simulink model "bh_SIM_7dof_car_active_suspension"  (R2022b)
settings: Solver=ode23t  StartTime=0.0  StopTime=10  FixedStep=0.0005  MaxStep=0.001  RelTol=1e-5
undefined symbols (not defined in the file): Continuous, K, OBJ_car_params, Time, X, Y, Z
libraries: sm_lib x23, nesl_utility x4, ctrlSharedLib x1
settings Model: Creator=bhorton  LastModifiedBy=bhorton
settings SolverCC: ZeroCrossAlgorithm=Adaptive
settings DebuggingCC: UnconnectedInputMsg=warning  UnconnectedOutputMsg=warning  UnconnectedLineMsg=warning
settings ModelReferenceCC: EnableRefExpFcnMdlSchedulingChecks=on
settings RTWCC: DLArmComputeVersion=19.05
settings ExplorerConfigSet: InternalSimMechanicsExplorerSettings="<ExplorerConfiguration><canonicalview>default</canonicalview><AnimationSetting><BasePlaybackSpeed>1.0</BasePlaybackSpeed><PlaybackSpeedFactor>1.0</PlaybackSpeedFactor></AnimationSetting><TilePanel><TileInfo><Tiles Columns=\"2\" Count=\"3\" Rows=\"2\"><Column Weight=\"0.4994\"/><Column Weight=\"0.5006\"/><Row Weight=\"0.4993\"/><Row Weight=\"0.5007\"/><Tile Height=\"1\" Width=\"2\" X=\"0\" Y=\"0\"/><Tile Height=\"1\" Width=\"1\" X=\"0\" Y=\"1\"/><Tile Height=\"1\" Width=\"1\" X=\"1\" Y=\"1\"/></Tiles></TileInfo><SceneInfo><SceneViewer><BGColor><R>0.60000002384185791</R><G>0.60000002384185791</G><B>0.60000002384185791</B></BGColor><Camera><DoPerspective>off</DoPerspective><Position><X>28.1684565527861146</X><Y>9.37690846949945644</Y><Z>23.0019248509705427</Z></Position><Center><X>8.88421556953053937</X><Y>0.438838580194179317</Y><Z>-4.64373243439162042</Z></Center><Up><X>-0.185673330126828295</X><Y>0.96548958646651295</Y><Z>-0.182634259941381938</Z></Up><ViewLimDist>1</ViewLimDist><YLim>3.64885946251190196</YLim><XLim>10.9300677112347469</XLim></Camera></SceneViewer><SceneViewer><BGColor><R>0.60000002384185791</R><G>0.60000002384185791</G><B>0.60000002384185791</B></BGColor><Camera><DoPerspective>off</DoPerspective><Position><X>5.74701636142130656</X><Y>11.5370316322497803</Y><Z>70.170564057313058</Z></Position><Center><X>1.87189459127800673</X><Y>1.93296934541278587</Y><Z>-0.938513511499806441</Z></Center><Up><X>-0.0228131350943184333</X><Y>0.990908416802929626</Y><Z>-0.132589857742894418</Z></Up><ViewLimDist>1</ViewLimDist><YLim>3.40641172776440104</YLim><XLim>5.04056870527299949</XLim></Camera></SceneViewer><SceneViewer><BGColor><R>0.60000002384185791</R><G>0.60000002384185791</G><B>0.60000002384185791</B></BGColor><Camera><DoPerspective>off</DoPerspective><Position><X>16.559571799394174</X><Y>1.27394383122949439</Y><Z>-2.29291646985018405</Z></Position><Center><X>1.86700752803715142</X><Y>-0.342587176142176597</Y><Z>-3.18464415250598165</Z></Center><Up><X>-0.109797444713875203</X><Y>0.993927323497863835</Y><Z>0.0072798858972461869</Z></Up><ViewLimDist>1</ViewLimDist><YLim>2.89568809729259158</YLim><XLim>4.29135758562730896</XLim></Camera></SceneViewer></SceneInfo></TilePanel><MechEditorPanel><Cameras/><GfxPanelCameraMap/><VideoCreator><PlaybackSpeedRatio>1.0</PlaybackSpeedRatio><FrameRate>30</FrameRate><VideoFormat>MPEG-4</VideoFormat><FrameSize>[400 400]</FrameSize></VideoCreator></MechEditorPanel></ExplorerConfiguration>"

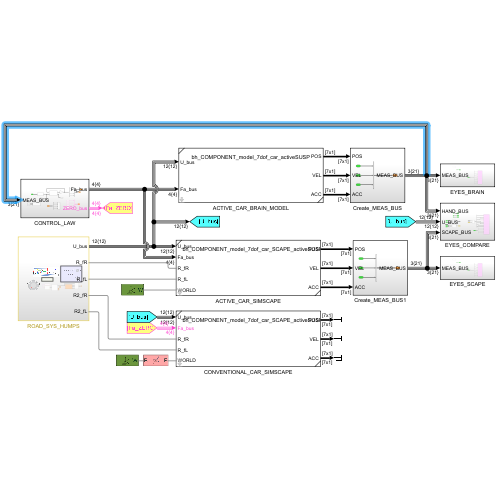
[thumbnail: Simulink's stored preview of the top-level diagram]
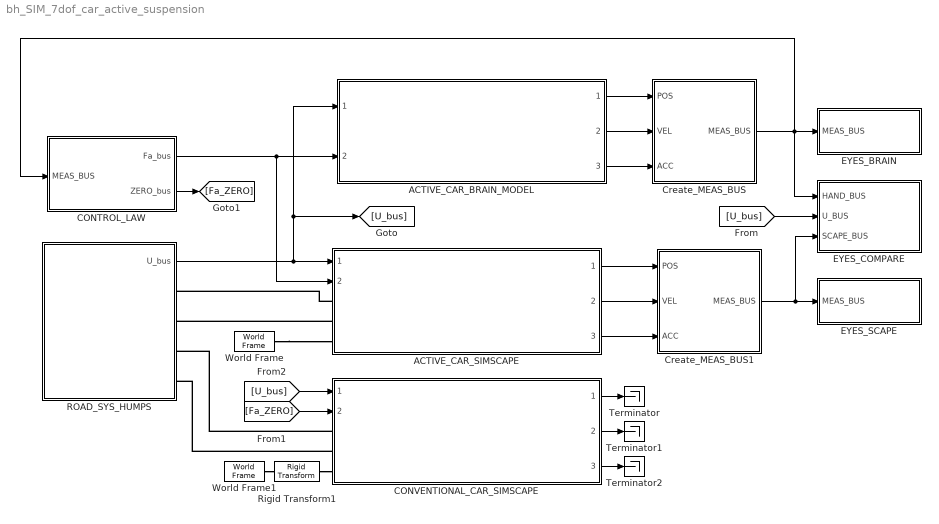
== system bh_SIM_7dof_car_active_suspension ==
  ACTIVE_CAR_BRAIN_MODEL : Subsystem  ReferencedSubsystem=bh_COMPONENT_model_7dof_car_activeSUSP  L_b=OBJ_car_params.L_b  L_f=OBJ_car_params.L_f  L_R=OBJ_car_params.L_R  L_L=OBJ_car_params.L_L  m_c=OBJ_car_params.m_c  I_cZ=OBJ_car_params.I_cZ  I_cX=OBJ_car_params.I_cX  m_bR=OBJ_car_params.m_bR  m_fR=OBJ_car_params.m_fR  m_bL=OBJ_car_params.m_bL  m_fL=OBJ_car_params.m_fL  k_bR=OBJ_car_params.k_bR  k_fR=OBJ_car_params.k_fR  k_bL=OBJ_car_params.k_bL  k_fL=OBJ_car_params.k_fL  k_bRG=OBJ_car_params.k_bRG  k_fRG=OBJ_car_params.k_fRG  k_bLG=OBJ_car_params.k_bLG  k_fLG=OBJ_car_params.k_fLG  c_bR=OBJ_car_params.c_bR  c_fR=OBJ_car_params.c_fR  c_bL=OBJ_car_params.c_bL  c_fL=OBJ_car_params.c_fL  c_bRG=OBJ_car_params.c_bRG  c_fRG=OBJ_car_params.c_fRG  c_bLG=OBJ_car_params.c_bLG  c_fLG=OBJ_car_params.c_fLG  IC_pos=OBJ_car_params.IC_pos  IC_vel=OBJ_car_params.IC_vel
  ACTIVE_CAR_SIMSCAPE : Subsystem  ReferencedSubsystem=bh_COMPONENT_model_7dof_car_SCAPE_activeSUSP  L_b=OBJ_car_params.L_b  L_f=OBJ_car_params.L_f  L_R=OBJ_car_params.L_R  L_L=OBJ_car_params.L_L  m_c=OBJ_car_params.m_c  I_cZ=OBJ_car_params.I_cZ  I_cX=OBJ_car_params.I_cX  m_bR=OBJ_car_params.m_bR  m_fR=OBJ_car_params.m_fR  m_bL=OBJ_car_params.m_bL  m_fL=OBJ_car_params.m_fL  k_bR=OBJ_car_params.k_bR  k_fR=OBJ_car_params.k_fR  k_bL=OBJ_car_params.k_bL  k_fL=OBJ_car_params.k_fL  k_bRG=OBJ_car_params.k_bRG  k_fRG=OBJ_car_params.k_fRG  k_bLG=OBJ_car_params.k_bLG  k_fLG=OBJ_car_params.k_fLG  c_bR=OBJ_car_params.c_bR  c_fR=OBJ_car_params.c_fR  c_bL=OBJ_car_params.c_bL  c_fL=OBJ_car_params.c_fL  c_bRG=OBJ_car_params.c_bRG  c_fRG=OBJ_car_params.c_fRG  c_bLG=OBJ_car_params.c_bLG  c_fLG=OBJ_car_params.c_fLG  IC_pos=OBJ_car_params.IC_pos  IC_vel=OBJ_car_params.IC_vel
  CONTROL_LAW : Subsystem
  CONVENTIONAL_CAR_SIMSCAPE : Subsystem  ReferencedSubsystem=bh_COMPONENT_model_7dof_car_SCAPE_activeSUSP  L_b=OBJ_car_params.L_b  L_f=OBJ_car_params.L_f  L_R=OBJ_car_params.L_R  L_L=OBJ_car_params.L_L  m_c=OBJ_car_params.m_c  I_cZ=OBJ_car_params.I_cZ  I_cX=OBJ_car_params.I_cX  m_bR=OBJ_car_params.m_bR  m_fR=OBJ_car_params.m_fR  m_bL=OBJ_car_params.m_bL  m_fL=OBJ_car_params.m_fL  k_bR=OBJ_car_params.k_bR  k_fR=OBJ_car_params.k_fR  k_bL=OBJ_car_params.k_bL  k_fL=OBJ_car_params.k_fL  k_bRG=OBJ_car_params.k_bRG  k_fRG=OBJ_car_params.k_fRG  k_bLG=OBJ_car_params.k_bLG  k_fLG=OBJ_car_params.k_fLG  c_bR=OBJ_car_params.c_bR  c_fR=OBJ_car_params.c_fR  c_bL=OBJ_car_params.c_bL  c_fL=OBJ_car_params.c_fL  c_bRG=OBJ_car_params.c_bRG  c_fRG=OBJ_car_params.c_fRG  c_bLG=OBJ_car_params.c_bLG  c_fLG=OBJ_car_params.c_fLG  IC_pos=OBJ_car_params.IC_pos  IC_vel=OBJ_car_params.IC_vel
  Create_MEAS_BUS : Subsystem
  Create_MEAS_BUS1 : Subsystem
  EYES_BRAIN : Subsystem
  EYES_COMPARE : Subsystem
  EYES_SCAPE : Subsystem
  ROAD_SYS_HUMPS : Subsystem
  Rigid Transform1 : sm_lib/Frames and Transforms/Rigid Transform  TranslationMethod=StandardAxis  TranslationStandardOffset=2*(OBJ_car_params.L_R + OBJ_car_params.L_L)  TranslationLengthUnit=m  TranslationStandardAxis=-Z  TranslationCartesianOffset=[0 0 0]  TranslationROffset=0  TranslationROffsetUnits=m  TranslationZOffset=0  TranslationZOffsetUnits=m  TranslationThetaOffset=0  TranslationThetaOffsetUnits=deg  RotationMethod=None  RotationAngleUnits=deg  RotationStandardAxis=+Z  RotationAngle=0.0  RotationArbitraryAxis=[0 0 1]  FollAlignAxisA=+X  BaseAlignAxisA=+Y  FollAlignAxisB=+Y  BaseAlignAxisB=+Z  RotationSequenceAxes=FollowerAxes  RotationSequence=XYX  RotationSequenceAngles=[0 0 0]  RotationSequenceAnglesUnits=deg  RotationMatrix=[1 0 0; 0 1 0; 0 0 1]  Quaternion=[1 0 0 0]
  Terminator : Terminator
  Terminator1 : Terminator
  Terminator2 : Terminator
  World Frame : sm_lib/Frames and Transforms/World Frame
  World Frame1 : sm_lib/Frames and Transforms/World Frame
  wires:
  ACTIVE_CAR_BRAIN_MODEL/1 -> Create_MEAS_BUS/1(POS)
  ACTIVE_CAR_BRAIN_MODEL/2 -> Create_MEAS_BUS/2(VEL)
  ACTIVE_CAR_BRAIN_MODEL/3 -> Create_MEAS_BUS/3(ACC)
  Create_MEAS_BUS/1(MEAS_BUS) -> EYES_COMPARE/1(HAND_BUS), CONTROL_LAW/1(MEAS_BUS), EYES_BRAIN/1(MEAS_BUS)
  ACTIVE_CAR_SIMSCAPE/1 -> Create_MEAS_BUS1/1(POS)
  ACTIVE_CAR_SIMSCAPE/2 -> Create_MEAS_BUS1/2(VEL)
  ACTIVE_CAR_SIMSCAPE/3 -> Create_MEAS_BUS1/3(ACC)
  Create_MEAS_BUS1/1(MEAS_BUS) -> EYES_COMPARE/3(SCAPE_BUS), EYES_SCAPE/1(MEAS_BUS)
  ROAD_SYS_HUMPS/1(U_bus) -> ACTIVE_CAR_BRAIN_MODEL/1, [U_bus], ACTIVE_CAR_SIMSCAPE/1
  [U_bus] -> EYES_COMPARE/2(U_BUS)
  CONTROL_LAW/2(ZERO_bus) -> [Fa_ZERO]
  CONTROL_LAW/1(Fa_bus) -> ACTIVE_CAR_SIMSCAPE/2, ACTIVE_CAR_BRAIN_MODEL/2
  [Fa_ZERO] -> CONVENTIONAL_CAR_SIMSCAPE/2
  [U_bus] -> CONVENTIONAL_CAR_SIMSCAPE/1
  CONVENTIONAL_CAR_SIMSCAPE/1 -> Terminator/1
  CONVENTIONAL_CAR_SIMSCAPE/2 -> Terminator1/1
  CONVENTIONAL_CAR_SIMSCAPE/3 -> Terminator2/1
  connections:
  ACTIVE_CAR_SIMSCAPE/LConn1 -- ROAD_SYS_HUMPS/RConn1
  ACTIVE_CAR_SIMSCAPE/LConn2 -- ROAD_SYS_HUMPS/RConn2
  World Frame1/RConn1 -- Rigid Transform1/LConn1
  Rigid Transform1/RConn1 -- CONVENTIONAL_CAR_SIMSCAPE/LConn3
  World Frame/RConn1 -- ACTIVE_CAR_SIMSCAPE/LConn3
  CONVENTIONAL_CAR_SIMSCAPE/LConn1 -- ROAD_SYS_HUMPS/RConn3
  CONVENTIONAL_CAR_SIMSCAPE/LConn2 -- ROAD_SYS_HUMPS/RConn4

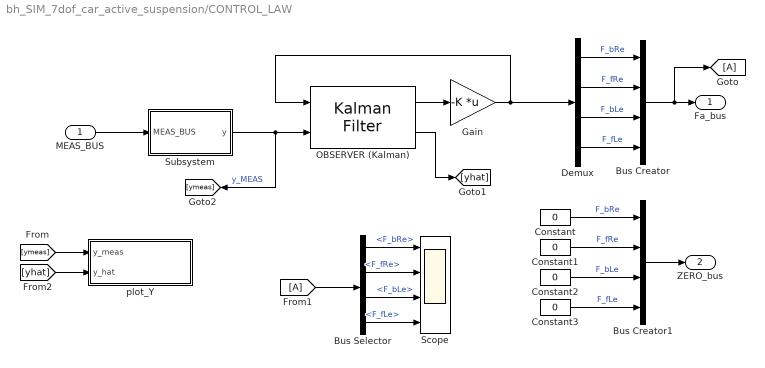
== system bh_SIM_7dof_car_active_suspension/CONTROL_LAW ==
  MEAS_BUS : Inport
  Bus Creator : BusCreator  Inputs=4
  Bus Creator1 : BusCreator  Inputs=4
  Bus Selector : BusSelector  OutputSignals=F_bRe,F_fRe,F_bLe,F_fLe
  Constant{,1..3} (4 alike) : Constant  Value=0
  Demux : Demux
  From1 : From
  Gain : Gain  Gain=-K  Multiplication=Matrix(K*u)
  Goto : Goto
  OBSERVER (Kalman) : ctrlSharedLib/Kalman Filter  TimeDomain=Continuous-Time  UseCurrentEstimator=on  ModelSource=LTI State-Space Variable  ModelSourceVariable=my_sys  A=0.95  B=1  C=1  D=0  NumberOfStates=1  NumberOfInputs=1  NumberOfOutputs=1  InitialEstimateSource=Dialog  X0=0  P0=10  UseK=off  UseGH=off  NumberOfProcessNoiseInputs=1  G=1  TimeInvariantG=on  H=0  TimeInvariantH=on  Q=1e8  TimeInvariantQ=on  R=1  TimeInvariantR=on  N=0  TimeInvariantN=on  AddInputPort=on  AddEnablePort=off  OutputEstimatedY=on  OutputP=off  Ts=-1
  Scope : Scope  NumInputPorts=4
  Subsystem : Subsystem
  plot_Y : Subsystem
  Fa_bus : Outport
  ZERO_bus : Outport  Port=2
  wires:
  MEAS_BUS/1 -> Subsystem/1(MEAS_BUS)
  Gain/1 -> OBSERVER (Kalman)/1, Demux/1
  Subsystem/1(y) -> [ymeas], OBSERVER (Kalman)/2  "y_MEAS"
  OBSERVER (Kalman)/1 -> Gain/1
  Demux/4 -> Bus Creator/4  "F_fLe"
  Demux/3 -> Bus Creator/3  "F_bLe"
  Demux/2 -> Bus Creator/2  "F_fRe"
  Demux/1 -> Bus Creator/1  "F_bRe"
  Bus Creator/1 -> Fa_bus/1, Goto/1
  From1/1 -> Bus Selector/1
  Bus Selector/1 -> Scope/1  "<F_bRe>"
  Bus Selector/2 -> Scope/2  "<F_fRe>"
  Bus Selector/3 -> Scope/3  "<F_bLe>"
  Bus Selector/4 -> Scope/4  "<F_fLe>"
  Bus Creator1/1 -> ZERO_bus/1
  Constant/1 -> Bus Creator1/1  "F_bRe"
  Constant3/1 -> Bus Creator1/4  "F_fLe"
  Constant2/1 -> Bus Creator1/3  "F_bLe"
  Constant1/1 -> Bus Creator1/2  "F_fRe"
  OBSERVER (Kalman)/2 -> [yhat]
  [ymeas] -> plot_Y/1(y_meas)
  [yhat] -> plot_Y/2(y_hat)

== system bh_SIM_7dof_car_active_suspension/Create_MEAS_BUS ==
  POS : Inport
  VEL : Inport  Port=2
  ACC : Inport  Port=3
  Bus Creator : BusCreator  Inputs=3
  MEAS_BUS : Outport
  wires:
  POS/1 -> Bus Creator/1  "POS"
  VEL/1 -> Bus Creator/2  "VEL"
  ACC/1 -> Bus Creator/3  "ACC"
  Bus Creator/1 -> MEAS_BUS/1

== system bh_SIM_7dof_car_active_suspension/Create_MEAS_BUS1 ==
  POS : Inport
  VEL : Inport  Port=2
  ACC : Inport  Port=3
  Bus Creator : BusCreator  Inputs=3
  MEAS_BUS : Outport
  wires:
  POS/1 -> Bus Creator/1  "POS"
  VEL/1 -> Bus Creator/2  "VEL"
  ACC/1 -> Bus Creator/3  "ACC"
  Bus Creator/1 -> MEAS_BUS/1

== system bh_SIM_7dof_car_active_suspension/EYES_BRAIN ==
  note: % NOTE:  the order of the DOF vector is:
      | %          1      2    3     4     5     6     7
      | %      [ y_c, theta, psi, y_bR, y_fR, y_bL, y_fL ]
  MEAS_BUS : Inport
  Bus Selector : BusSelector  OutputSignals=POS
  Demux : Demux  Outputs=7
  Ground : Ground
  HAND_POS : Scope  NumInputPorts=8
  Subsystem : Subsystem  Commented=on
  wires:
  MEAS_BUS/1 -> [MEAS]
  Demux/1 -> HAND_POS/1  "y_c"
  Demux/2 -> HAND_POS/2  "theta"
  Demux/3 -> HAND_POS/3  "psi"
  Ground/1 -> HAND_POS/4
  Demux/4 -> HAND_POS/5  "y_bR"
  Demux/5 -> HAND_POS/6  "y_fR"
  Demux/6 -> HAND_POS/7  "y_bL"
  Demux/7 -> HAND_POS/8  "y_fL"
  [MEAS] -> Bus Selector/1
  Bus Selector/1 -> Demux/1  "<POS>"

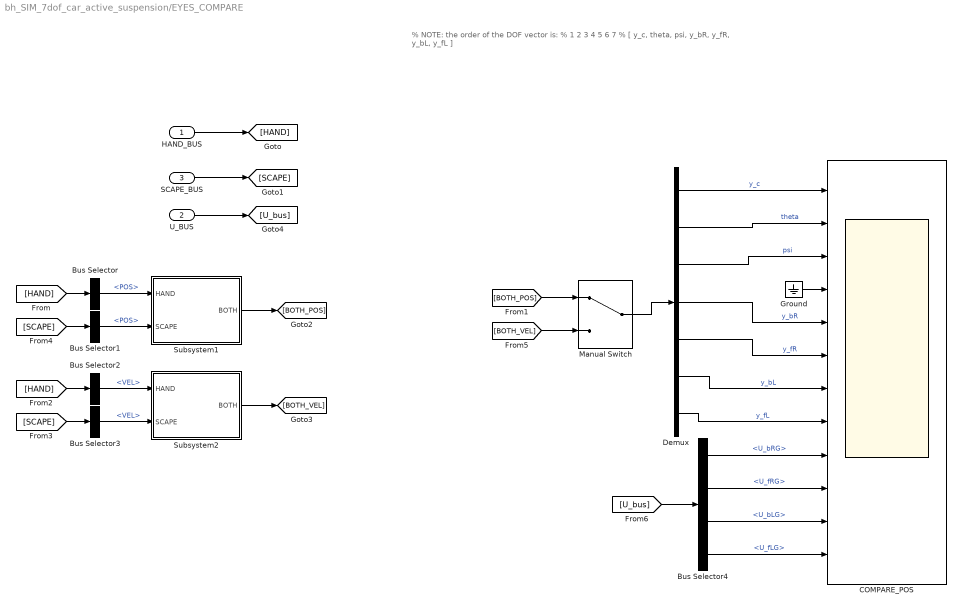
== system bh_SIM_7dof_car_active_suspension/EYES_COMPARE ==
  note: % NOTE:  the order of the DOF vector is:
      | %          1      2    3     4     5     6     7
      | %      [ y_c, theta, psi, y_bR, y_fR, y_bL, y_fL ]
  HAND_BUS : Inport
  U_BUS : Inport  Port=2
  SCAPE_BUS : Inport  Port=3
  Bus Selector : BusSelector  OutputSignals=POS
  Bus Selector1 : BusSelector  OutputSignals=POS
  Bus Selector2 : BusSelector  OutputSignals=VEL
  Bus Selector3 : BusSelector  OutputSignals=VEL
  Bus Selector4 : BusSelector  OutputSignals=U_bRG,U_fRG,U_bLG,U_fLG
  COMPARE_POS : Scope  NumInputPorts=12
  Demux : Demux  Outputs=7
  Ground : Ground
  Manual Switch : ManualSwitch
  Subsystem1 : Subsystem
  Subsystem2 : Subsystem
  wires:
  HAND_BUS/1 -> [HAND]
  Demux/1 -> COMPARE_POS/1  "y_c"
  Demux/2 -> COMPARE_POS/2  "theta"
  Demux/3 -> COMPARE_POS/3  "psi"
  Ground/1 -> COMPARE_POS/4
  Demux/5 -> COMPARE_POS/6  "y_fR"
  Demux/6 -> COMPARE_POS/7  "y_bL"
  Demux/7 -> COMPARE_POS/8  "y_fL"
  SCAPE_BUS/1 -> [SCAPE]
  [HAND] -> Bus Selector/1
  [SCAPE] -> Bus Selector1/1
  Bus Selector/1 -> Subsystem1/1(HAND)  "<POS>"
  Bus Selector1/1 -> Subsystem1/2(SCAPE)  "<POS>"
  Subsystem1/1(BOTH) -> [BOTH_POS]
  [HAND] -> Bus Selector2/1
  Subsystem2/1(BOTH) -> [BOTH_VEL]
  Bus Selector2/1 -> Subsystem2/1(HAND)  "<VEL>"
  Bus Selector3/1 -> Subsystem2/2(SCAPE)  "<VEL>"
  [SCAPE] -> Bus Selector3/1
  Manual Switch/1 -> Demux/1
  [BOTH_VEL] -> Manual Switch/2
  [BOTH_POS] -> Manual Switch/1
  U_BUS/1 -> [U_bus]
  [U_bus] -> Bus Selector4/1
  Bus Selector4/4 -> COMPARE_POS/12  "<U_fLG>"
  Bus Selector4/3 -> COMPARE_POS/11  "<U_bLG>"
  Bus Selector4/2 -> COMPARE_POS/10  "<U_fRG>"
  Bus Selector4/1 -> COMPARE_POS/9  "<U_bRG>"
  Demux/4 -> COMPARE_POS/5  "y_bR"

== system bh_SIM_7dof_car_active_suspension/EYES_SCAPE ==
  note: % NOTE:  the order of the DOF vector is:
      | %          1      2    3     4     5     6     7
      | %      [ y_c, theta, psi, y_bR, y_fR, y_bL, y_fL ]
  MEAS_BUS : Inport
  Bus Selector : BusSelector  OutputSignals=POS
  Demux : Demux  Outputs=7
  Ground : Ground
  SCAPE_POS : Scope  NumInputPorts=8
  Subsystem : Subsystem  Commented=on
  wires:
  MEAS_BUS/1 -> [MEAS]
  Demux/1 -> SCAPE_POS/1  "y_c"
  Demux/2 -> SCAPE_POS/2  "theta"
  Demux/3 -> SCAPE_POS/3  "psi"
  Ground/1 -> SCAPE_POS/4
  Demux/4 -> SCAPE_POS/5  "y_bR"
  Demux/5 -> SCAPE_POS/6  "y_fR"
  Demux/6 -> SCAPE_POS/7  "y_bL"
  Demux/7 -> SCAPE_POS/8  "y_fL"
  [MEAS] -> Bus Selector/1
  Bus Selector/1 -> Demux/1  "<POS>"

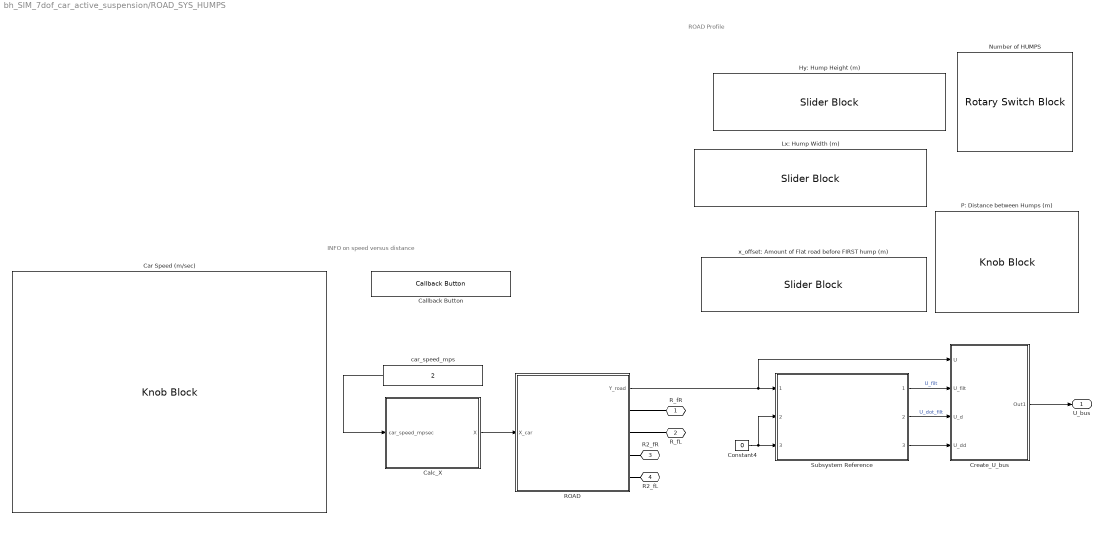
== system bh_SIM_7dof_car_active_suspension/ROAD_SYS_HUMPS ==
  note: INFO on speed versus distance
  note: ROAD Profile
  Calc_X : Subsystem
  Callback Button : CallbackButton  ButtonText=Open XLS file to view
      settings: ClickFcn=winopen bh_speed_vs_distance_explore.xlsx
  Car Speed (m/sec) : KnobBlock  LabelPosition=Hide  ScaleMax=30  TickInterval=1
  Constant4 : Constant  Value=0
  Create_U_bus : Subsystem
  Hy: Hump Height (m) : SliderBlock  LabelPosition=Hide  ScaleMax=0.16
  Lx: Hump Width (m) : SliderBlock  LabelPosition=Hide  ScaleMax=1
  Number of HUMPS : RotarySwitchBlock  LabelPosition=Hide
      settings: Values={{'1', '3', '5', '10', '20', '50', '100'}, [1 3 5 10 20 50 100]}
  P: Distance between Humps (m) : KnobBlock  LabelPosition=Hide
  ROAD : Subsystem  mask{m_Hy=0.16, m_Lx=1, m_P=2, m_x_offset=2, m_Np=5}
      mask prompts: m_Hy "Height of hump (m)"; m_Lx "Length of hump (m)"; m_P "Period of window (m)"; m_x_offset "X direction offset"; m_Np "Number of periods"
      mask init:
      | % create SYS object
      | OBJ = bh_road_hump_A_SYSO("Hy",m_Hy, "Lx",m_Lx, "P",m_P, ...
      |                           "x_offset",m_x_offset, "NUM_PERIODS",m_Np);
      |                       
      | tmp_x = linspace(0,(m_Np*m_P  +  m_x_offset), 1e4);
      | tmp_y = OBJ.get_y(tmp_x);
      | %tmp_z = -2 * ones(size(tmp_x));
      | tmp_z = zeros(size(tmp_x));
      | the_road_XYZ = [ tmp_x(:), tmp_y(:), tmp_z(:) ];
      mask DialogControl Control2 Prompt: Road Profile Parameters
      mask DialogControl Container6 Prompt: Road Profile Parameters
  Subsystem Reference : Subsystem  ReferencedSubsystem=bh_COMPONENT_deriv_est  wn=2*pi*5000  p=1
  car_speed_mps : Constant  Value=2
  x_offset: Amount of Flat road before FIRST hump (m) : SliderBlock  LabelPosition=Hide  ScaleMax=10
  R_fR : PMIOPort  Side=Right
  R_fL : PMIOPort  Port=2  Side=Right
  R2_fR : PMIOPort  Port=3  Side=Right
  R2_fL : PMIOPort  Port=4  Side=Right
  U_bus : Outport
  wires:
  Create_U_bus/1(Out1) -> U_bus/1
  ROAD/1(Y_road) -> Create_U_bus/1(U), Subsystem Reference/1
  Constant4/1 -> Subsystem Reference/2, Subsystem Reference/3
  Subsystem Reference/3 -> Create_U_bus/4(U_dd)
  Subsystem Reference/2 -> Create_U_bus/3(U_d)  "U_dot_filt"
  Subsystem Reference/1 -> Create_U_bus/2(U_filt)  "U_filt"
  Calc_X/1(X) -> ROAD/1(X_car)
  car_speed_mps/1 -> Calc_X/1(car_speed_mpsec)
  connections:
  R_fL/RConn1 -- ROAD/RConn2
  ROAD/RConn1 -- R_fR/RConn1
  ROAD/RConn3 -- R2_fR/RConn1
  ROAD/RConn4 -- R2_fL/RConn1

== system bh_SIM_7dof_car_active_suspension/CONTROL_LAW/Subsystem ==
  note: $X^T =\left\lbrack \begin{array}{ccccccc} y_c & \theta & \psi & y_{\mathrm{bR}} & y_{\mathrm{fR}} & y_{\mathrm{bL}} & y_{\mathrm{fL}} \end{array}\right\rbrack \\ Z=\left\lbrack \begin{array}{c} \dot{X} \\ X \end{array}\right\rbrack \\ y={\left\lbrack \begin{array}{cccccc} y_c & \theta & \psi & \dot{y_c } & \dot{\theta} & \dot{\psi} \end{array}\right\rbrack }^T$
  MEAS_BUS : Inport
  Bus Selector : BusSelector  OutputSignals=VEL,POS
  Constant4 : Constant  Value="[8,9,10,  1,2,3]"
  Selector : Selector  InputPortWidth=14  IndexOptions=Index vector (port)  Indices=[1 3]  OutputSizes=1
  Vector Concatenate : Concatenate
  y : Outport
  wires:
  Bus Selector/1 -> Vector Concatenate/1  "<VEL>"
  MEAS_BUS/1 -> Bus Selector/1
  Bus Selector/2 -> Vector Concatenate/2  "<POS>"
  Constant4/1 -> Selector/2  "F_fLe"
  Vector Concatenate/1 -> Selector/1  "Z"
  Selector/1 -> y/1

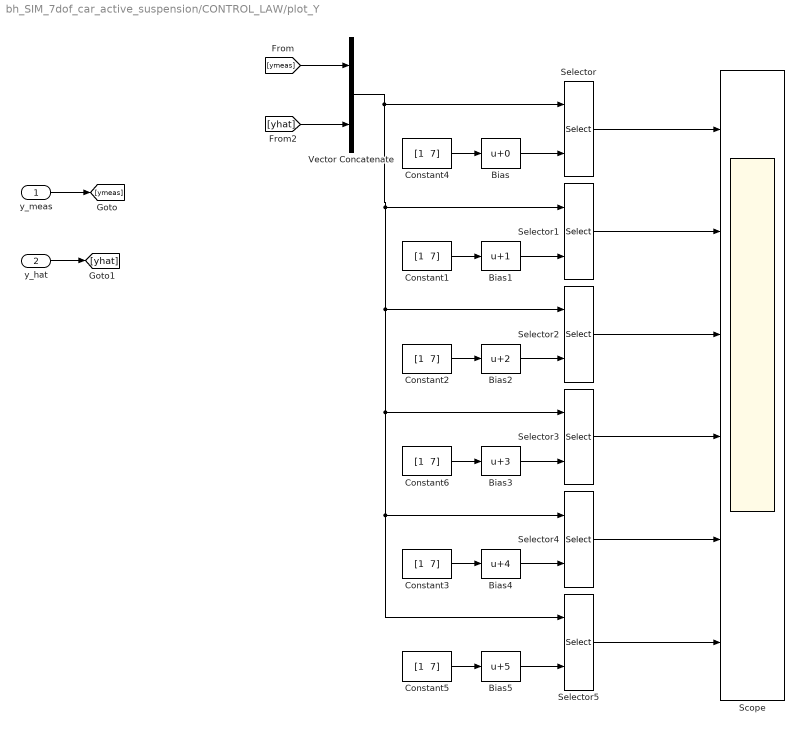
== system bh_SIM_7dof_car_active_suspension/CONTROL_LAW/plot_Y ==
  y_meas : Inport
  y_hat : Inport  Port=2
  Bias : Bias  SaturateOnIntegerOverflow=off
  Bias1 : Bias  Bias=1  SaturateOnIntegerOverflow=off
  Bias2 : Bias  Bias=2  SaturateOnIntegerOverflow=off
  Bias3 : Bias  Bias=3  SaturateOnIntegerOverflow=off
  Bias4 : Bias  Bias=4  SaturateOnIntegerOverflow=off
  Bias5 : Bias  Bias=5  SaturateOnIntegerOverflow=off
  Constant{1..6} (6 alike) : Constant  Value="[1  7]"
  Scope : Scope  NumInputPorts=6
  Selector{,1..5} (6 alike) : Selector  InputPortWidth=12  IndexOptions=Index vector (port)  Indices=[1 3]  OutputSizes=1
  Vector Concatenate : Concatenate
  wires:
  y_meas/1 -> [ymeas]
  y_hat/1 -> [yhat]
  [ymeas] -> Vector Concatenate/1
  [yhat] -> Vector Concatenate/2
  Constant4/1 -> Bias/1
  Bias/1 -> Selector/2
  Selector/1 -> Scope/1
  Bias1/1 -> Selector1/2
  Constant1/1 -> Bias1/1
  Selector1/1 -> Scope/2
  Bias2/1 -> Selector2/2
  Constant2/1 -> Bias2/1
  Selector2/1 -> Scope/3
  Bias3/1 -> Selector3/2
  Constant3/1 -> Bias4/1
  Bias4/1 -> Selector4/2
  Vector Concatenate/1 -> Selector3/1, Selector5/1, Selector4/1, Selector2/1, Selector1/1, Selector/1
  Constant6/1 -> Bias3/1
  Bias5/1 -> Selector5/2
  Constant5/1 -> Bias5/1
  Selector3/1 -> Scope/4
  Selector4/1 -> Scope/5
  Selector5/1 -> Scope/6

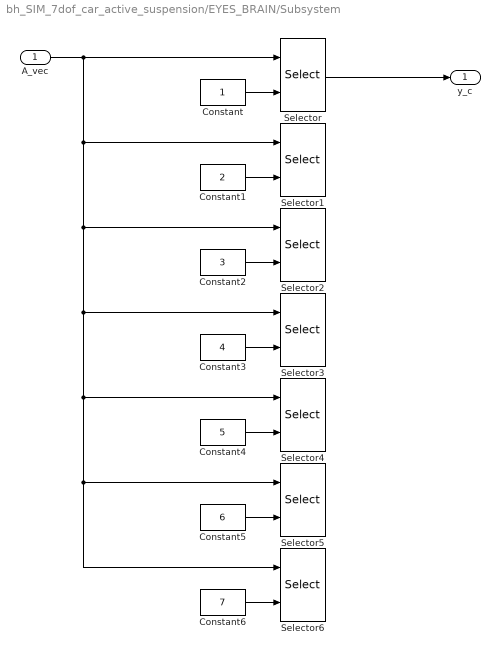
== system bh_SIM_7dof_car_active_suspension/EYES_BRAIN/Subsystem ==
  A_vec : Inport
  Constant : Constant
  Constant1 : Constant  Value=2
  Constant2 : Constant  Value=3
  Constant3 : Constant  Value=4
  Constant4 : Constant  Value=5
  Constant5 : Constant  Value=6
  Constant6 : Constant  Value=7
  Selector{,1..6} (7 alike) : Selector  InputPortWidth=7  IndexOptions=Index vector (port)  Indices=1  OutputSizes=1
  y_c : Outport
  wires:
  Constant/1 -> Selector/2
  Constant1/1 -> Selector1/2
  Constant2/1 -> Selector2/2
  Constant3/1 -> Selector3/2
  Constant4/1 -> Selector4/2
  Constant5/1 -> Selector5/2
  Constant6/1 -> Selector6/2
  A_vec/1 -> Selector1/1, Selector2/1, Selector3/1, Selector4/1, Selector5/1, Selector6/1, Selector/1
  Selector/1 -> y_c/1

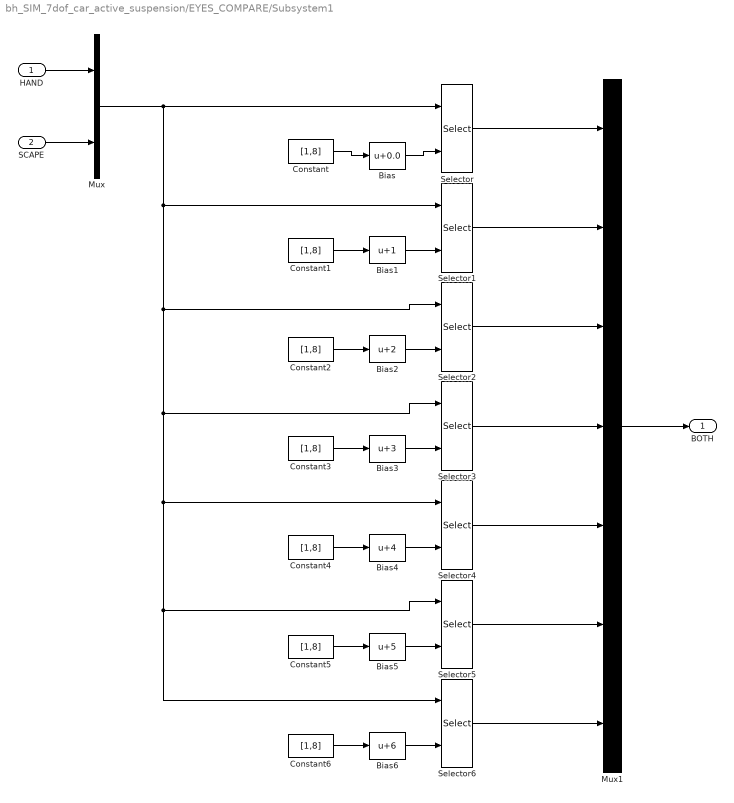
== system bh_SIM_7dof_car_active_suspension/EYES_COMPARE/Subsystem1 ==
  HAND : Inport
  SCAPE : Inport  Port=2
  Bias : Bias  Bias=0.0  SaturateOnIntegerOverflow=off
  Bias1 : Bias  Bias=1  SaturateOnIntegerOverflow=off
  Bias2 : Bias  Bias=2  SaturateOnIntegerOverflow=off
  Bias3 : Bias  Bias=3  SaturateOnIntegerOverflow=off
  Bias4 : Bias  Bias=4  SaturateOnIntegerOverflow=off
  Bias5 : Bias  Bias=5  SaturateOnIntegerOverflow=off
  Bias6 : Bias  Bias=6  SaturateOnIntegerOverflow=off
  Constant{,1..6} (7 alike) : Constant  Value=[1,8]
  Mux : Mux  Inputs=2
  Mux1 : Mux  Inputs=7
  Selector{,1..6} (7 alike) : Selector  InputPortWidth=14  IndexOptions=Index vector (port)  Indices=[1 3]  OutputSizes=1
  BOTH : Outport
  wires:
  SCAPE/1 -> Mux/2
  HAND/1 -> Mux/1
  Constant/1 -> Bias/1
  Bias/1 -> Selector/2
  Selector/1 -> Mux1/1
  Selector1/1 -> Mux1/2
  Bias1/1 -> Selector1/2
  Constant1/1 -> Bias1/1
  Constant2/1 -> Bias2/1
  Bias2/1 -> Selector2/2
  Selector2/1 -> Mux1/3
  Bias3/1 -> Selector3/2
  Constant3/1 -> Bias3/1
  Selector3/1 -> Mux1/4
  Constant4/1 -> Bias4/1
  Bias4/1 -> Selector4/2
  Selector4/1 -> Mux1/5
  Constant5/1 -> Bias5/1
  Bias5/1 -> Selector5/2
  Constant6/1 -> Bias6/1
  Bias6/1 -> Selector6/2
  Mux/1 -> Selector1/1, Selector2/1, Selector3/1, Selector4/1, Selector5/1, Selector6/1, Selector/1
  Selector5/1 -> Mux1/6
  Selector6/1 -> Mux1/7
  Mux1/1 -> BOTH/1

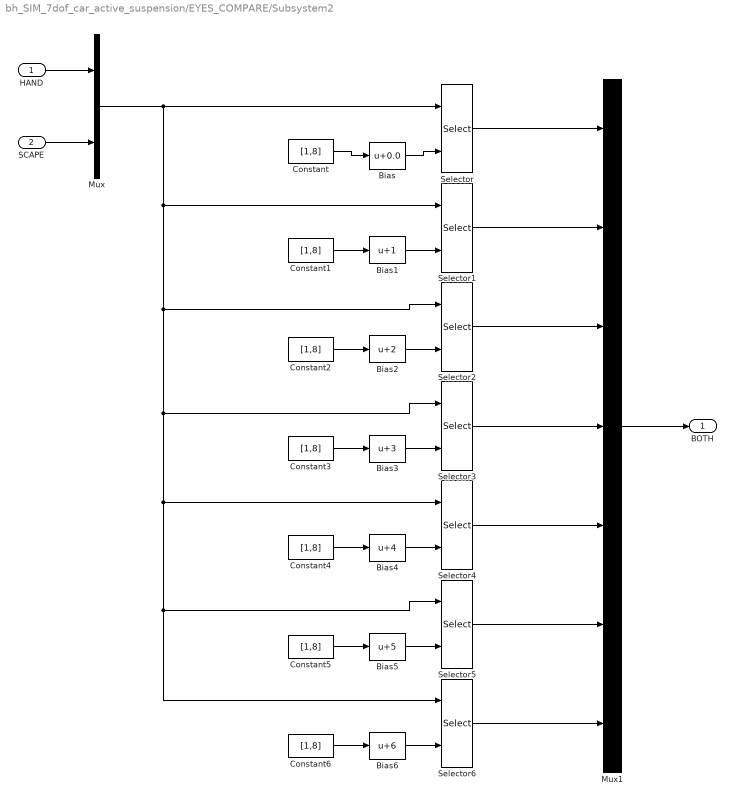
== system bh_SIM_7dof_car_active_suspension/EYES_COMPARE/Subsystem2 ==
  HAND : Inport
  SCAPE : Inport  Port=2
  Bias : Bias  Bias=0.0  SaturateOnIntegerOverflow=off
  Bias1 : Bias  Bias=1  SaturateOnIntegerOverflow=off
  Bias2 : Bias  Bias=2  SaturateOnIntegerOverflow=off
  Bias3 : Bias  Bias=3  SaturateOnIntegerOverflow=off
  Bias4 : Bias  Bias=4  SaturateOnIntegerOverflow=off
  Bias5 : Bias  Bias=5  SaturateOnIntegerOverflow=off
  Bias6 : Bias  Bias=6  SaturateOnIntegerOverflow=off
  Constant{,1..6} (7 alike) : Constant  Value=[1,8]
  Mux : Mux  Inputs=2
  Mux1 : Mux  Inputs=7
  Selector{,1..6} (7 alike) : Selector  InputPortWidth=14  IndexOptions=Index vector (port)  Indices=[1 3]  OutputSizes=1
  BOTH : Outport
  wires:
  SCAPE/1 -> Mux/2
  HAND/1 -> Mux/1
  Constant/1 -> Bias/1
  Bias/1 -> Selector/2
  Selector/1 -> Mux1/1
  Selector1/1 -> Mux1/2
  Bias1/1 -> Selector1/2
  Constant1/1 -> Bias1/1
  Constant2/1 -> Bias2/1
  Bias2/1 -> Selector2/2
  Selector2/1 -> Mux1/3
  Bias3/1 -> Selector3/2
  Constant3/1 -> Bias3/1
  Selector3/1 -> Mux1/4
  Constant4/1 -> Bias4/1
  Bias4/1 -> Selector4/2
  Selector4/1 -> Mux1/5
  Constant5/1 -> Bias5/1
  Bias5/1 -> Selector5/2
  Constant6/1 -> Bias6/1
  Bias6/1 -> Selector6/2
  Mux/1 -> Selector1/1, Selector2/1, Selector3/1, Selector4/1, Selector5/1, Selector6/1, Selector/1
  Selector5/1 -> Mux1/6
  Selector6/1 -> Mux1/7
  Mux1/1 -> BOTH/1

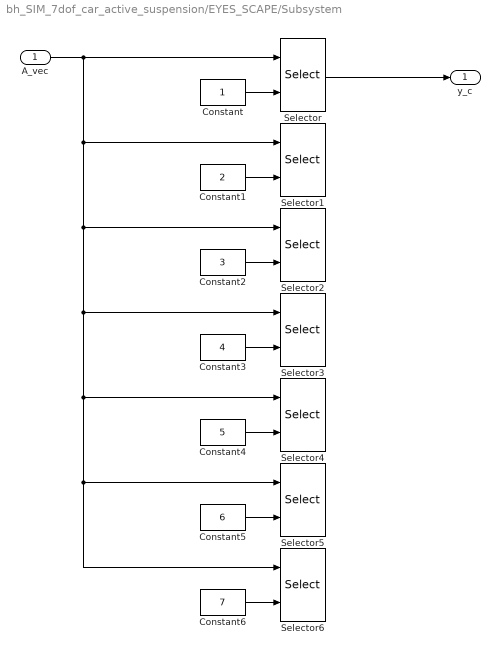
== system bh_SIM_7dof_car_active_suspension/EYES_SCAPE/Subsystem ==
  A_vec : Inport
  Constant : Constant
  Constant1 : Constant  Value=2
  Constant2 : Constant  Value=3
  Constant3 : Constant  Value=4
  Constant4 : Constant  Value=5
  Constant5 : Constant  Value=6
  Constant6 : Constant  Value=7
  Selector{,1..6} (7 alike) : Selector  InputPortWidth=7  IndexOptions=Index vector (port)  Indices=1  OutputSizes=1
  y_c : Outport
  wires:
  Constant/1 -> Selector/2
  Constant1/1 -> Selector1/2
  Constant2/1 -> Selector2/2
  Constant3/1 -> Selector3/2
  Constant4/1 -> Selector4/2
  Constant5/1 -> Selector5/2
  Constant6/1 -> Selector6/2
  A_vec/1 -> Selector1/1, Selector2/1, Selector3/1, Selector4/1, Selector5/1, Selector6/1, Selector/1
  Selector/1 -> y_c/1

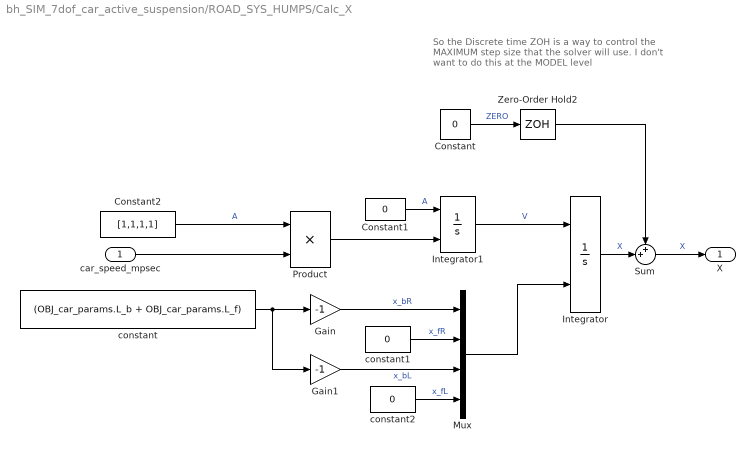
== system bh_SIM_7dof_car_active_suspension/ROAD_SYS_HUMPS/Calc_X ==
  note: So the Discrete time ZOH is a way to control
      | the MAXIMUM step size that the solver will use.
      |
      | I don't want to do this at the MODEL level
  car_speed_mpsec : Inport
  Constant : Constant  Value=0
  Constant1 : Constant  Value=0
  Constant2 : Constant  Value=[1,1,1,1]
  Gain : Gain  Gain=-1
  Gain1 : Gain  Gain=-1
  Integrator : Integrator  InitialConditionSource=external
  Integrator1 : Integrator  InitialConditionSource=external
  Mux : Mux
  Product : Product
  Sum : Sum  Inputs=++|
  Zero-Order Hold2 : ZeroOrderHold  SampleTime=1/1000
      settings: AttributesFormatString=dT =%<SampleTime>
  constant : Constant  Value=(OBJ_car_params.L_b + OBJ_car_params.L_f)
  constant1 : Constant  Value=0
  constant2 : Constant  Value=0
  X : Outport
  wires:
  Integrator1/1 -> Integrator/1  "V"
  Zero-Order Hold2/1 -> Sum/1
  car_speed_mpsec/1 -> Product/2
  Integrator/1 -> Sum/2  "X"
  Constant/1 -> Zero-Order Hold2/1  "ZERO"
  Mux/1 -> Integrator/2
  Constant1/1 -> Integrator1/1  "A"
  constant/1 -> Gain1/1, Gain/1
  constant2/1 -> Mux/4  "x_fL"
  Gain1/1 -> Mux/3  "x_bL"
  constant1/1 -> Mux/2  "x_fR"
  Gain/1 -> Mux/1  "x_bR"
  Sum/1 -> X/1  "X"
  Constant2/1 -> Product/1  "A"
  Product/1 -> Integrator1/2

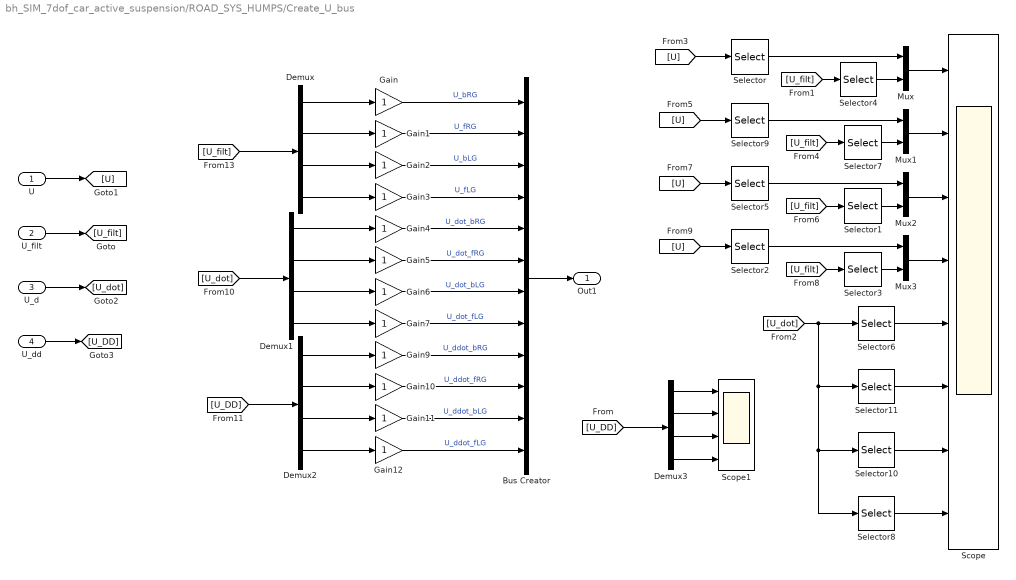
== system bh_SIM_7dof_car_active_suspension/ROAD_SYS_HUMPS/Create_U_bus ==
  U : Inport
  U_filt : Inport  Port=2
  U_d : Inport  Port=3
  U_dd : Inport  Port=4
  Bus Creator : BusCreator  Inputs=12
  Demux{,1..3} (4 alike) : Demux
  Gain{,1..7,9..12} (12 alike) : Gain
  Mux{,1..3} (4 alike) : Mux  Inputs=2
  Scope : Scope  NumInputPorts=8
  Scope1 : Scope  NumInputPorts=4
  Selector : Selector  InputPortWidth=4  IndexOptions=Index vector (dialog)  Indices=1  OutputSizes=1
  Selector1 : Selector  InputPortWidth=4  IndexOptions=Index vector (dialog)  Indices=3  OutputSizes=1
  Selector10 : Selector  InputPortWidth=4  IndexOptions=Index vector (dialog)  Indices=3  OutputSizes=1
  Selector11 : Selector  InputPortWidth=4  IndexOptions=Index vector (dialog)  Indices=2  OutputSizes=1
  Selector2 : Selector  InputPortWidth=4  IndexOptions=Index vector (dialog)  Indices=4  OutputSizes=1
  Selector3 : Selector  InputPortWidth=4  IndexOptions=Index vector (dialog)  Indices=4  OutputSizes=1
  Selector4 : Selector  InputPortWidth=4  IndexOptions=Index vector (dialog)  Indices=1  OutputSizes=1
  Selector5 : Selector  InputPortWidth=4  IndexOptions=Index vector (dialog)  Indices=3  OutputSizes=1
  Selector6 : Selector  InputPortWidth=4  IndexOptions=Index vector (dialog)  Indices=1  OutputSizes=1
  Selector7 : Selector  InputPortWidth=4  IndexOptions=Index vector (dialog)  Indices=2  OutputSizes=1
  Selector8 : Selector  InputPortWidth=4  IndexOptions=Index vector (dialog)  Indices=4  OutputSizes=1
  Selector9 : Selector  InputPortWidth=4  IndexOptions=Index vector (dialog)  Indices=2  OutputSizes=1
  Out1 : Outport
  wires:
  Demux/1 -> Gain/1
  [U_dot] -> Selector11/1, Selector10/1, Selector8/1, Selector6/1
  Gain9/1 -> Bus Creator/9  "U_ddot_bRG"
  Gain10/1 -> Bus Creator/10  "U_ddot_fRG"
  Gain1/1 -> Bus Creator/2  "U_fRG"
  Demux/2 -> Gain1/1
  Mux/1 -> Scope/1
  Demux/3 -> Gain2/1
  Demux2/2 -> Gain10/1
  Demux1/4 -> Gain7/1
  Demux3/3 -> Scope1/3
  Gain4/1 -> Bus Creator/5  "U_dot_bRG"
  Demux1/2 -> Gain5/1
  Demux1/3 -> Gain6/1
  Selector6/1 -> Scope/5
  Gain7/1 -> Bus Creator/8  "U_dot_fLG"
  Demux2/1 -> Gain9/1
  Gain5/1 -> Bus Creator/6  "U_dot_fRG"
  Demux1/1 -> Gain4/1
  [U_filt] -> Selector1/1
  Selector3/1 -> Mux3/2
  Gain2/1 -> Bus Creator/3  "U_bLG"
  Demux/4 -> Gain3/1
  [U] -> Selector2/1
  Gain3/1 -> Bus Creator/4  "U_fLG"
  Selector10/1 -> Scope/7
  Selector7/1 -> Mux1/2
  Selector4/1 -> Mux/2
  Selector11/1 -> Scope/6
  Gain/1 -> Bus Creator/1  "U_bRG"
  Mux2/1 -> Scope/3
  Mux1/1 -> Scope/2
  Mux3/1 -> Scope/4
  Selector5/1 -> Mux2/1
  [U] -> Selector/1
  Selector8/1 -> Scope/8
  Gain6/1 -> Bus Creator/7  "U_dot_bLG"
  Selector2/1 -> Mux3/1
  [U] -> Selector5/1
  Selector1/1 -> Mux2/2
  Selector9/1 -> Mux1/1
  Demux3/2 -> Scope1/2
  [U_filt] -> Selector4/1
  [U_filt] -> Selector7/1
  Selector/1 -> Mux/1
  Demux3/1 -> Scope1/1
  Gain12/1 -> Bus Creator/12  "U_ddot_fLG"
  [U] -> Selector9/1
  Bus Creator/1 -> Out1/1
  Demux3/4 -> Scope1/4
  Demux2/4 -> Gain12/1
  [U_DD] -> Demux3/1
  Gain11/1 -> Bus Creator/11  "U_ddot_bLG"
  [U_filt] -> Selector3/1
  Demux2/3 -> Gain11/1
  U/1 -> [U]
  U_filt/1 -> [U_filt]
  U_d/1 -> [U_dot]
  U_dd/1 -> [U_DD]
  [U_dot] -> Demux1/1
  [U_DD] -> Demux2/1
  [U_filt] -> Demux/1

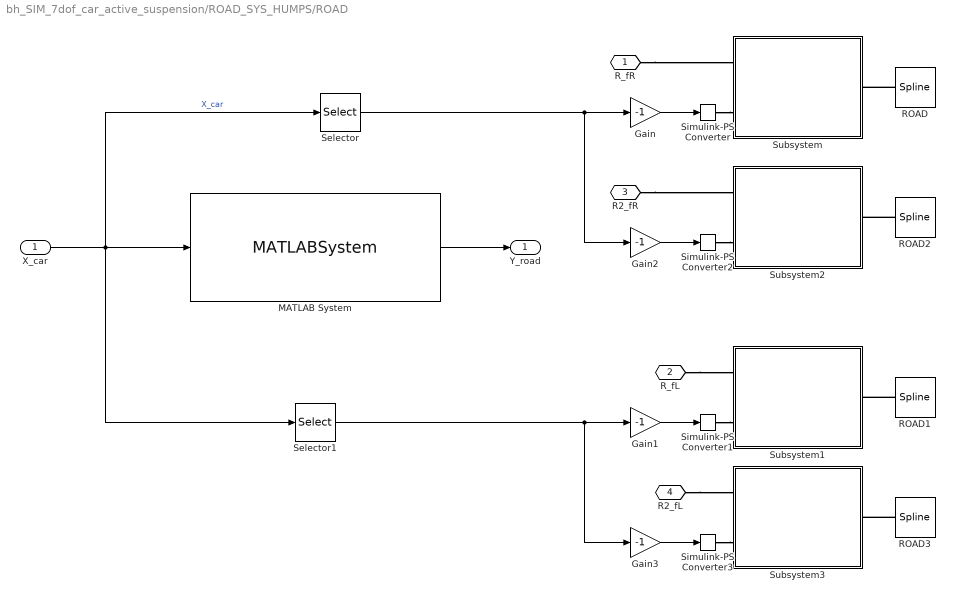
== system bh_SIM_7dof_car_active_suspension/ROAD_SYS_HUMPS/ROAD ==
  X_car : Inport
  Gain{,1..3} (4 alike) : Gain  Gain=-1
  MATLAB System : MATLABSystem  System=bh_road_hump_A_SYSO  Hy=m_Hy  Lx=m_Lx  P=m_P  x_offset=m_x_offset  NUM_PERIODS=m_Np  SimulateUsing=Interpreted execution
      mask Type: bh_road_hump_A_SYSO
      mask Display:
      | disp('bh_road_hump_A_SYSO');
      | port_label('input',1,'X_car');
      | port_label('output',1,'Y_road');
  ROAD : sm_lib/Curves and Surfaces/Spline  GraphicAmbientColor=[0.15 0.15 0.15 1.0]  GraphicDiffuseColor=[0.2 1.0 0.2]  DataPoints=the_road_XYZ  DataPointsUnits=m  GraphicEmissiveColor=[0.0 0.0 0.0 1.0]  EndConditionType=Natural  MarkerShape=Sphere  MarkerSize=10  GraphicType=FromGeometry  GraphicOpacity=1.0  GraphicShininess=75  GraphicSpecularColor=[0.5 0.5 0.5 1.0]  GraphicVisPropType=SimpleVisualProperties
  ROAD1 : sm_lib/Curves and Surfaces/Spline  GraphicAmbientColor=[0.15 0.15 0.15 1.0]  GraphicDiffuseColor=[0.2 1.0 0.2]  DataPoints=the_road_XYZ  DataPointsUnits=m  GraphicEmissiveColor=[0.0 0.0 0.0 1.0]  EndConditionType=Natural  MarkerShape=Sphere  MarkerSize=10  GraphicType=FromGeometry  GraphicOpacity=1.0  GraphicShininess=75  GraphicSpecularColor=[0.5 0.5 0.5 1.0]  GraphicVisPropType=SimpleVisualProperties
  ROAD2 : sm_lib/Curves and Surfaces/Spline  GraphicAmbientColor=[0.15 0.15 0.15 1.0]  GraphicDiffuseColor=[1, 0.6, 0.6]  DataPoints=the_road_XYZ  DataPointsUnits=m  GraphicEmissiveColor=[0.0 0.0 0.0 1.0]  EndConditionType=Natural  MarkerShape=Sphere  MarkerSize=10  GraphicType=FromGeometry  GraphicOpacity=1.0  GraphicShininess=75  GraphicSpecularColor=[0.5 0.5 0.5 1.0]  GraphicVisPropType=SimpleVisualProperties
  ROAD3 : sm_lib/Curves and Surfaces/Spline  GraphicAmbientColor=[0.15 0.15 0.15 1.0]  GraphicDiffuseColor=[1.0 0.6 0.6]  DataPoints=the_road_XYZ  DataPointsUnits=m  GraphicEmissiveColor=[0.0 0.0 0.0 1.0]  EndConditionType=Natural  MarkerShape=Sphere  MarkerSize=10  GraphicType=FromGeometry  GraphicOpacity=1.0  GraphicShininess=75  GraphicSpecularColor=[0.5 0.5 0.5 1.0]  GraphicVisPropType=SimpleVisualProperties
  Selector : Selector  InputPortWidth=4  IndexOptions=Index vector (dialog)  Indices=2  OutputSizes=1
  Selector1 : Selector  InputPortWidth=4  IndexOptions=Index vector (dialog)  Indices=4  OutputSizes=1
  Simulink-PS Converter{,1..3} (4 alike) : nesl_utility/Simulink-PS Converter  PhysicalDomain=network_engine_domain  SubClassName=ps_input  LeftPortType=input  RightPortType=output  PseudoPeriodic=off  Frequencies=[]  NoiseDistribution=none  NoiseParameters=[]  Unit=m  AffineConversion=off  FilteringAndDerivatives=filter  SimscapeFilterOrder=2  InputFilterTimeConstant=0.001  UdotUserProvided=0
  Subsystem : Subsystem
  Subsystem1 : Subsystem
  Subsystem2 : Subsystem
  Subsystem3 : Subsystem
  R_fR : PMIOPort  Side=Right
  R_fL : PMIOPort  Port=2  Side=Right
  R2_fR : PMIOPort  Port=3  Side=Right
  R2_fL : PMIOPort  Port=4  Side=Right
  Y_road : Outport
  wires:
  MATLAB System/1 -> Y_road/1
  X_car/1 -> Selector1/1, Selector/1, MATLAB System/1  "X_car"
  Selector/1 -> Gain2/1, Gain/1
  Gain/1 -> Simulink-PS Converter/1
  Gain1/1 -> Simulink-PS Converter1/1
  Gain2/1 -> Simulink-PS Converter2/1
  Gain3/1 -> Simulink-PS Converter3/1
  Selector1/1 -> Gain1/1, Gain3/1
  connections:
  Simulink-PS Converter/RConn1 -- Subsystem/LConn2
  ROAD/LConn1 -- Subsystem/RConn1
  R_fR/RConn1 -- Subsystem/LConn1
  Simulink-PS Converter1/RConn1 -- Subsystem1/LConn2
  ROAD1/LConn1 -- Subsystem1/RConn1
  R_fL/RConn1 -- Subsystem1/LConn1
  R2_fR/RConn1 -- Subsystem2/LConn1
  Simulink-PS Converter2/RConn1 -- Subsystem2/LConn2
  ROAD2/LConn1 -- Subsystem2/RConn1
  R2_fL/RConn1 -- Subsystem3/LConn1
  ROAD3/LConn1 -- Subsystem3/RConn1
  Simulink-PS Converter3/RConn1 -- Subsystem3/LConn2

== system bh_SIM_7dof_car_active_suspension/ROAD_SYS_HUMPS/ROAD/Subsystem ==
  Prismatic Joint2 : sm_lib/Joints/Prismatic Joint  JointMode=Normal  SenseConstraintForce=off  SenseConstraintForceX=off  SenseConstraintForceY=off  SenseConstraintForceZ=off  SenseConstraintTorque=off  SenseConstraintTorqueX=off  SenseConstraintTorqueY=off  SenseConstraintTorqueZ=off  SenseTotalForce=off  SenseTotalForceX=off  SenseTotalForceY=off  SenseTotalForceZ=off  SenseTotalTorque=off  SenseTotalTorqueX=off  SenseTotalTorqueY=off  SenseTotalTorqueZ=off  CompositeWrenchDir=FollowerOnBase  CompositeWrenchFrame=BaseFrame  EquilibriumPosition=0  EquilibriumPositionUnits=m  SpringStiffness=0  SpringStiffnessUnits=N/m  DampingCoefficient=0  DampingCoefficientUnits=N/(m/s)  TorqueActuationMode=ComputedTorque  MotionActuationMode=InputMotion  SensePosition=off  SenseVelocity=off  SenseAcceleration=off  SenseTorqueForce=off  SenseLowerLimitTorqueForce=off  SenseUpperLimitTorqueForce=off  LowerLimitSpecify=off  LowerLimitBound=-1  LowerLimitBoundUnits=m  LowerLimitStiffness=1e6  LowerLimitStiffnessUnits=N/m  LowerLimitDamping=1e3  LowerLimitDampingUnits=N/(m/s)  LowerLimitTransitionRegionWidth=1e-4  LowerLimitTransitionRegionWidthUnits=m  UpperLimitSpecify=off  UpperLimitBound=1  UpperLimitBoundUnits=m  UpperLimitStiffness=1e6  UpperLimitStiffnessUnits=N/m  UpperLimitDamping=1e3  UpperLimitDampingUnits=N/(m/s)  UpperLimitTransitionRegionWidth=1e-4  UpperLimitTransitionRegionWidthUnits=m  PositionTargetSpecify=off  PositionTargetPriority=High  PositionTargetValue=0  PositionTargetValueUnits=m  VelocityTargetSpecify=off  VelocityTargetPriority=High  VelocityTargetValue=0  VelocityTargetValueUnits=m/s
  ROAD_CARRIER_MASS : sm_lib/Body Elements/Brick Solid  GraphicAmbientColor=[0.15 0.15 0.15 1.0]  BasedOnType=Density  BrickDimensions=[1, 1, 1]/100  BrickDimensionUnits=m  CenterOfMass=[0 0 0]  CenterOfMassUnits=m  GraphicDiffuseColor=[0.0 0.8 0.2]  Density=1000  DensityUnits=kg/m^3  DoExposeReferenceFrame=on  GraphicEmissiveColor=[0.0 0.0 0.0 1.0]  ExportEntireGeometry=off  SerializedFrames=<Frames/>  MarkerShape=Sphere  MarkerSize=10  GraphicType=FromGeometry  InertiaType=PointMass  Mass=1  MassUnits=kg  MomentsOfInertia=[1 1 1]  MomentsOfInertiaUnits=kg*m^2  GraphicOpacity=1.0  ProductsOfInertia=[0 0 0]  ProductsOfInertiaUnits=kg*m^2  GraphicShininess=75  GraphicSpecularColor=[0.5 0.5 0.5 1.0]  GraphicVisPropType=SimpleVisualProperties
  Rigid Transform4 : sm_lib/Frames and Transforms/Rigid Transform  TranslationMethod=None  TranslationStandardOffset=0  TranslationLengthUnit=m  TranslationStandardAxis=+Z  TranslationCartesianOffset=[0 0 0]  TranslationROffset=0  TranslationROffsetUnits=m  TranslationZOffset=0  TranslationZOffsetUnits=m  TranslationThetaOffset=0  TranslationThetaOffsetUnits=deg  RotationMethod=AlignedAxes  RotationAngleUnits=deg  RotationStandardAxis=+Z  RotationAngle=0.0  RotationArbitraryAxis=[0 0 1]  FollAlignAxisA=+Z  BaseAlignAxisA=+X  FollAlignAxisB=+Y  BaseAlignAxisB=+Y  RotationSequenceAxes=FollowerAxes  RotationSequence=XYX  RotationSequenceAngles=[0 0 0]  RotationSequenceAnglesUnits=deg  RotationMatrix=[1 0 0; 0 1 0; 0 0 1]  Quaternion=[1 0 0 0]
  Rigid Transform5 : sm_lib/Frames and Transforms/Rigid Transform  TranslationMethod=None  TranslationStandardOffset=0  TranslationLengthUnit=m  TranslationStandardAxis=+Z  TranslationCartesianOffset=[0 0 0]  TranslationROffset=0  TranslationROffsetUnits=m  TranslationZOffset=0  TranslationZOffsetUnits=m  TranslationThetaOffset=0  TranslationThetaOffsetUnits=deg  RotationMethod=AlignedAxes  RotationAngleUnits=deg  RotationStandardAxis=+Z  RotationAngle=0.0  RotationArbitraryAxis=[0 0 1]  FollAlignAxisA=+X  BaseAlignAxisA=+Z  FollAlignAxisB=+Y  BaseAlignAxisB=+Y  RotationSequenceAxes=FollowerAxes  RotationSequence=XYX  RotationSequenceAngles=[0 0 0]  RotationSequenceAnglesUnits=deg  RotationMatrix=[1 0 0; 0 1 0; 0 0 1]  Quaternion=[1 0 0 0]
  XY_F_Origin : PMIOPort  Side=Left
  RMASS : PMIOPort  Port=2  Side=Right
  POS_NEG_RMASS : PMIOPort  Port=3  Side=Left
  connections:
  Prismatic Joint2/LConn1 -- Rigid Transform4/RConn1
  Rigid Transform5/LConn1 -- Prismatic Joint2/RConn1
  Prismatic Joint2/LConn2 -- POS_NEG_RMASS/RConn1
  Rigid Transform4/LConn1 -- XY_F_Origin/RConn1
  Rigid Transform5/RConn1 -- ROAD_CARRIER_MASS/RConn1 -- RMASS/RConn1

== system bh_SIM_7dof_car_active_suspension/ROAD_SYS_HUMPS/ROAD/Subsystem1 ==
  Prismatic Joint2 : sm_lib/Joints/Prismatic Joint  JointMode=Normal  SenseConstraintForce=off  SenseConstraintForceX=off  SenseConstraintForceY=off  SenseConstraintForceZ=off  SenseConstraintTorque=off  SenseConstraintTorqueX=off  SenseConstraintTorqueY=off  SenseConstraintTorqueZ=off  SenseTotalForce=off  SenseTotalForceX=off  SenseTotalForceY=off  SenseTotalForceZ=off  SenseTotalTorque=off  SenseTotalTorqueX=off  SenseTotalTorqueY=off  SenseTotalTorqueZ=off  CompositeWrenchDir=FollowerOnBase  CompositeWrenchFrame=BaseFrame  EquilibriumPosition=0  EquilibriumPositionUnits=m  SpringStiffness=0  SpringStiffnessUnits=N/m  DampingCoefficient=0  DampingCoefficientUnits=N/(m/s)  TorqueActuationMode=ComputedTorque  MotionActuationMode=InputMotion  SensePosition=off  SenseVelocity=off  SenseAcceleration=off  SenseTorqueForce=off  SenseLowerLimitTorqueForce=off  SenseUpperLimitTorqueForce=off  LowerLimitSpecify=off  LowerLimitBound=-1  LowerLimitBoundUnits=m  LowerLimitStiffness=1e6  LowerLimitStiffnessUnits=N/m  LowerLimitDamping=1e3  LowerLimitDampingUnits=N/(m/s)  LowerLimitTransitionRegionWidth=1e-4  LowerLimitTransitionRegionWidthUnits=m  UpperLimitSpecify=off  UpperLimitBound=1  UpperLimitBoundUnits=m  UpperLimitStiffness=1e6  UpperLimitStiffnessUnits=N/m  UpperLimitDamping=1e3  UpperLimitDampingUnits=N/(m/s)  UpperLimitTransitionRegionWidth=1e-4  UpperLimitTransitionRegionWidthUnits=m  PositionTargetSpecify=off  PositionTargetPriority=High  PositionTargetValue=0  PositionTargetValueUnits=m  VelocityTargetSpecify=off  VelocityTargetPriority=High  VelocityTargetValue=0  VelocityTargetValueUnits=m/s
  ROAD_CARRIER_MASS : sm_lib/Body Elements/Brick Solid  GraphicAmbientColor=[0.15 0.15 0.15 1.0]  BasedOnType=Density  BrickDimensions=[1, 1, 1]/100  BrickDimensionUnits=m  CenterOfMass=[0 0 0]  CenterOfMassUnits=m  GraphicDiffuseColor=[0.0 0.8 0.2]  Density=1000  DensityUnits=kg/m^3  DoExposeReferenceFrame=on  GraphicEmissiveColor=[0.0 0.0 0.0 1.0]  ExportEntireGeometry=off  SerializedFrames=<Frames/>  MarkerShape=Sphere  MarkerSize=10  GraphicType=FromGeometry  InertiaType=PointMass  Mass=1  MassUnits=kg  MomentsOfInertia=[1 1 1]  MomentsOfInertiaUnits=kg*m^2  GraphicOpacity=1.0  ProductsOfInertia=[0 0 0]  ProductsOfInertiaUnits=kg*m^2  GraphicShininess=75  GraphicSpecularColor=[0.5 0.5 0.5 1.0]  GraphicVisPropType=SimpleVisualProperties
  Rigid Transform4 : sm_lib/Frames and Transforms/Rigid Transform  TranslationMethod=None  TranslationStandardOffset=0  TranslationLengthUnit=m  TranslationStandardAxis=+Z  TranslationCartesianOffset=[0 0 0]  TranslationROffset=0  TranslationROffsetUnits=m  TranslationZOffset=0  TranslationZOffsetUnits=m  TranslationThetaOffset=0  TranslationThetaOffsetUnits=deg  RotationMethod=AlignedAxes  RotationAngleUnits=deg  RotationStandardAxis=+Z  RotationAngle=0.0  RotationArbitraryAxis=[0 0 1]  FollAlignAxisA=+Z  BaseAlignAxisA=+X  FollAlignAxisB=+Y  BaseAlignAxisB=+Y  RotationSequenceAxes=FollowerAxes  RotationSequence=XYX  RotationSequenceAngles=[0 0 0]  RotationSequenceAnglesUnits=deg  RotationMatrix=[1 0 0; 0 1 0; 0 0 1]  Quaternion=[1 0 0 0]
  Rigid Transform5 : sm_lib/Frames and Transforms/Rigid Transform  TranslationMethod=None  TranslationStandardOffset=0  TranslationLengthUnit=m  TranslationStandardAxis=+Z  TranslationCartesianOffset=[0 0 0]  TranslationROffset=0  TranslationROffsetUnits=m  TranslationZOffset=0  TranslationZOffsetUnits=m  TranslationThetaOffset=0  TranslationThetaOffsetUnits=deg  RotationMethod=AlignedAxes  RotationAngleUnits=deg  RotationStandardAxis=+Z  RotationAngle=0.0  RotationArbitraryAxis=[0 0 1]  FollAlignAxisA=+X  BaseAlignAxisA=+Z  FollAlignAxisB=+Y  BaseAlignAxisB=+Y  RotationSequenceAxes=FollowerAxes  RotationSequence=XYX  RotationSequenceAngles=[0 0 0]  RotationSequenceAnglesUnits=deg  RotationMatrix=[1 0 0; 0 1 0; 0 0 1]  Quaternion=[1 0 0 0]
  XY_F_Origin : PMIOPort  Side=Left
  RMASS : PMIOPort  Port=2  Side=Right
  POS_NEG_RMASS : PMIOPort  Port=3  Side=Left
  connections:
  Prismatic Joint2/LConn1 -- Rigid Transform4/RConn1
  Rigid Transform5/LConn1 -- Prismatic Joint2/RConn1
  Prismatic Joint2/LConn2 -- POS_NEG_RMASS/RConn1
  Rigid Transform4/LConn1 -- XY_F_Origin/RConn1
  Rigid Transform5/RConn1 -- ROAD_CARRIER_MASS/RConn1 -- RMASS/RConn1

== system bh_SIM_7dof_car_active_suspension/ROAD_SYS_HUMPS/ROAD/Subsystem2 ==
  Prismatic Joint2 : sm_lib/Joints/Prismatic Joint  JointMode=Normal  SenseConstraintForce=off  SenseConstraintForceX=off  SenseConstraintForceY=off  SenseConstraintForceZ=off  SenseConstraintTorque=off  SenseConstraintTorqueX=off  SenseConstraintTorqueY=off  SenseConstraintTorqueZ=off  SenseTotalForce=off  SenseTotalForceX=off  SenseTotalForceY=off  SenseTotalForceZ=off  SenseTotalTorque=off  SenseTotalTorqueX=off  SenseTotalTorqueY=off  SenseTotalTorqueZ=off  CompositeWrenchDir=FollowerOnBase  CompositeWrenchFrame=BaseFrame  EquilibriumPosition=0  EquilibriumPositionUnits=m  SpringStiffness=0  SpringStiffnessUnits=N/m  DampingCoefficient=0  DampingCoefficientUnits=N/(m/s)  TorqueActuationMode=ComputedTorque  MotionActuationMode=InputMotion  SensePosition=off  SenseVelocity=off  SenseAcceleration=off  SenseTorqueForce=off  SenseLowerLimitTorqueForce=off  SenseUpperLimitTorqueForce=off  LowerLimitSpecify=off  LowerLimitBound=-1  LowerLimitBoundUnits=m  LowerLimitStiffness=1e6  LowerLimitStiffnessUnits=N/m  LowerLimitDamping=1e3  LowerLimitDampingUnits=N/(m/s)  LowerLimitTransitionRegionWidth=1e-4  LowerLimitTransitionRegionWidthUnits=m  UpperLimitSpecify=off  UpperLimitBound=1  UpperLimitBoundUnits=m  UpperLimitStiffness=1e6  UpperLimitStiffnessUnits=N/m  UpperLimitDamping=1e3  UpperLimitDampingUnits=N/(m/s)  UpperLimitTransitionRegionWidth=1e-4  UpperLimitTransitionRegionWidthUnits=m  PositionTargetSpecify=off  PositionTargetPriority=High  PositionTargetValue=0  PositionTargetValueUnits=m  VelocityTargetSpecify=off  VelocityTargetPriority=High  VelocityTargetValue=0  VelocityTargetValueUnits=m/s
  ROAD_CARRIER_MASS : sm_lib/Body Elements/Brick Solid  GraphicAmbientColor=[0.15 0.15 0.15 1.0]  BasedOnType=Density  BrickDimensions=[1, 1, 1]/100  BrickDimensionUnits=m  CenterOfMass=[0 0 0]  CenterOfMassUnits=m  GraphicDiffuseColor=[0.0 0.8 0.2]  Density=1000  DensityUnits=kg/m^3  DoExposeReferenceFrame=on  GraphicEmissiveColor=[0.0 0.0 0.0 1.0]  ExportEntireGeometry=off  SerializedFrames=<Frames/>  MarkerShape=Sphere  MarkerSize=10  GraphicType=FromGeometry  InertiaType=PointMass  Mass=1  MassUnits=kg  MomentsOfInertia=[1 1 1]  MomentsOfInertiaUnits=kg*m^2  GraphicOpacity=1.0  ProductsOfInertia=[0 0 0]  ProductsOfInertiaUnits=kg*m^2  GraphicShininess=75  GraphicSpecularColor=[0.5 0.5 0.5 1.0]  GraphicVisPropType=SimpleVisualProperties
  Rigid Transform4 : sm_lib/Frames and Transforms/Rigid Transform  TranslationMethod=None  TranslationStandardOffset=0  TranslationLengthUnit=m  TranslationStandardAxis=+Z  TranslationCartesianOffset=[0 0 0]  TranslationROffset=0  TranslationROffsetUnits=m  TranslationZOffset=0  TranslationZOffsetUnits=m  TranslationThetaOffset=0  TranslationThetaOffsetUnits=deg  RotationMethod=AlignedAxes  RotationAngleUnits=deg  RotationStandardAxis=+Z  RotationAngle=0.0  RotationArbitraryAxis=[0 0 1]  FollAlignAxisA=+Z  BaseAlignAxisA=+X  FollAlignAxisB=+Y  BaseAlignAxisB=+Y  RotationSequenceAxes=FollowerAxes  RotationSequence=XYX  RotationSequenceAngles=[0 0 0]  RotationSequenceAnglesUnits=deg  RotationMatrix=[1 0 0; 0 1 0; 0 0 1]  Quaternion=[1 0 0 0]
  Rigid Transform5 : sm_lib/Frames and Transforms/Rigid Transform  TranslationMethod=None  TranslationStandardOffset=0  TranslationLengthUnit=m  TranslationStandardAxis=+Z  TranslationCartesianOffset=[0 0 0]  TranslationROffset=0  TranslationROffsetUnits=m  TranslationZOffset=0  TranslationZOffsetUnits=m  TranslationThetaOffset=0  TranslationThetaOffsetUnits=deg  RotationMethod=AlignedAxes  RotationAngleUnits=deg  RotationStandardAxis=+Z  RotationAngle=0.0  RotationArbitraryAxis=[0 0 1]  FollAlignAxisA=+X  BaseAlignAxisA=+Z  FollAlignAxisB=+Y  BaseAlignAxisB=+Y  RotationSequenceAxes=FollowerAxes  RotationSequence=XYX  RotationSequenceAngles=[0 0 0]  RotationSequenceAnglesUnits=deg  RotationMatrix=[1 0 0; 0 1 0; 0 0 1]  Quaternion=[1 0 0 0]
  XY_F_Origin : PMIOPort  Side=Left
  RMASS : PMIOPort  Port=2  Side=Right
  POS_NEG_RMASS : PMIOPort  Port=3  Side=Left
  connections:
  Prismatic Joint2/LConn1 -- Rigid Transform4/RConn1
  Rigid Transform5/LConn1 -- Prismatic Joint2/RConn1
  Prismatic Joint2/LConn2 -- POS_NEG_RMASS/RConn1
  Rigid Transform4/LConn1 -- XY_F_Origin/RConn1
  Rigid Transform5/RConn1 -- ROAD_CARRIER_MASS/RConn1 -- RMASS/RConn1

== system bh_SIM_7dof_car_active_suspension/ROAD_SYS_HUMPS/ROAD/Subsystem3 ==
  Prismatic Joint2 : sm_lib/Joints/Prismatic Joint  JointMode=Normal  SenseConstraintForce=off  SenseConstraintForceX=off  SenseConstraintForceY=off  SenseConstraintForceZ=off  SenseConstraintTorque=off  SenseConstraintTorqueX=off  SenseConstraintTorqueY=off  SenseConstraintTorqueZ=off  SenseTotalForce=off  SenseTotalForceX=off  SenseTotalForceY=off  SenseTotalForceZ=off  SenseTotalTorque=off  SenseTotalTorqueX=off  SenseTotalTorqueY=off  SenseTotalTorqueZ=off  CompositeWrenchDir=FollowerOnBase  CompositeWrenchFrame=BaseFrame  EquilibriumPosition=0  EquilibriumPositionUnits=m  SpringStiffness=0  SpringStiffnessUnits=N/m  DampingCoefficient=0  DampingCoefficientUnits=N/(m/s)  TorqueActuationMode=ComputedTorque  MotionActuationMode=InputMotion  SensePosition=off  SenseVelocity=off  SenseAcceleration=off  SenseTorqueForce=off  SenseLowerLimitTorqueForce=off  SenseUpperLimitTorqueForce=off  LowerLimitSpecify=off  LowerLimitBound=-1  LowerLimitBoundUnits=m  LowerLimitStiffness=1e6  LowerLimitStiffnessUnits=N/m  LowerLimitDamping=1e3  LowerLimitDampingUnits=N/(m/s)  LowerLimitTransitionRegionWidth=1e-4  LowerLimitTransitionRegionWidthUnits=m  UpperLimitSpecify=off  UpperLimitBound=1  UpperLimitBoundUnits=m  UpperLimitStiffness=1e6  UpperLimitStiffnessUnits=N/m  UpperLimitDamping=1e3  UpperLimitDampingUnits=N/(m/s)  UpperLimitTransitionRegionWidth=1e-4  UpperLimitTransitionRegionWidthUnits=m  PositionTargetSpecify=off  PositionTargetPriority=High  PositionTargetValue=0  PositionTargetValueUnits=m  VelocityTargetSpecify=off  VelocityTargetPriority=High  VelocityTargetValue=0  VelocityTargetValueUnits=m/s
  ROAD_CARRIER_MASS : sm_lib/Body Elements/Brick Solid  GraphicAmbientColor=[0.15 0.15 0.15 1.0]  BasedOnType=Density  BrickDimensions=[1, 1, 1]/100  BrickDimensionUnits=m  CenterOfMass=[0 0 0]  CenterOfMassUnits=m  GraphicDiffuseColor=[0.0 0.8 0.2]  Density=1000  DensityUnits=kg/m^3  DoExposeReferenceFrame=on  GraphicEmissiveColor=[0.0 0.0 0.0 1.0]  ExportEntireGeometry=off  SerializedFrames=<Frames/>  MarkerShape=Sphere  MarkerSize=10  GraphicType=FromGeometry  InertiaType=PointMass  Mass=1  MassUnits=kg  MomentsOfInertia=[1 1 1]  MomentsOfInertiaUnits=kg*m^2  GraphicOpacity=1.0  ProductsOfInertia=[0 0 0]  ProductsOfInertiaUnits=kg*m^2  GraphicShininess=75  GraphicSpecularColor=[0.5 0.5 0.5 1.0]  GraphicVisPropType=SimpleVisualProperties
  Rigid Transform4 : sm_lib/Frames and Transforms/Rigid Transform  TranslationMethod=None  TranslationStandardOffset=0  TranslationLengthUnit=m  TranslationStandardAxis=+Z  TranslationCartesianOffset=[0 0 0]  TranslationROffset=0  TranslationROffsetUnits=m  TranslationZOffset=0  TranslationZOffsetUnits=m  TranslationThetaOffset=0  TranslationThetaOffsetUnits=deg  RotationMethod=AlignedAxes  RotationAngleUnits=deg  RotationStandardAxis=+Z  RotationAngle=0.0  RotationArbitraryAxis=[0 0 1]  FollAlignAxisA=+Z  BaseAlignAxisA=+X  FollAlignAxisB=+Y  BaseAlignAxisB=+Y  RotationSequenceAxes=FollowerAxes  RotationSequence=XYX  RotationSequenceAngles=[0 0 0]  RotationSequenceAnglesUnits=deg  RotationMatrix=[1 0 0; 0 1 0; 0 0 1]  Quaternion=[1 0 0 0]
  Rigid Transform5 : sm_lib/Frames and Transforms/Rigid Transform  TranslationMethod=None  TranslationStandardOffset=0  TranslationLengthUnit=m  TranslationStandardAxis=+Z  TranslationCartesianOffset=[0 0 0]  TranslationROffset=0  TranslationROffsetUnits=m  TranslationZOffset=0  TranslationZOffsetUnits=m  TranslationThetaOffset=0  TranslationThetaOffsetUnits=deg  RotationMethod=AlignedAxes  RotationAngleUnits=deg  RotationStandardAxis=+Z  RotationAngle=0.0  RotationArbitraryAxis=[0 0 1]  FollAlignAxisA=+X  BaseAlignAxisA=+Z  FollAlignAxisB=+Y  BaseAlignAxisB=+Y  RotationSequenceAxes=FollowerAxes  RotationSequence=XYX  RotationSequenceAngles=[0 0 0]  RotationSequenceAnglesUnits=deg  RotationMatrix=[1 0 0; 0 1 0; 0 0 1]  Quaternion=[1 0 0 0]
  XY_F_Origin : PMIOPort  Side=Left
  RMASS : PMIOPort  Port=2  Side=Right
  POS_NEG_RMASS : PMIOPort  Port=3  Side=Left
  connections:
  Prismatic Joint2/LConn1 -- Rigid Transform4/RConn1
  Rigid Transform5/LConn1 -- Prismatic Joint2/RConn1
  Prismatic Joint2/LConn2 -- POS_NEG_RMASS/RConn1
  Rigid Transform4/LConn1 -- XY_F_Origin/RConn1
  Rigid Transform5/RConn1 -- ROAD_CARRIER_MASS/RConn1 -- RMASS/RConn1
